simulink model "discrete_angular_rate_subsystem_eso"  (R2019b)
settings: Solver=FixedStepAuto  StartTime=0.0  StopTime=50  FixedStep=1/sim_freq  RelTol=1e-3
values from neighbouring files (symbols this model uses):
  A = diag(ones(length(a)-2,1),1)    [eso_design.m]    (also in eso_design_angular_rate.m = [0 1 0; 0 0 1; 0 0 -500 ]; eso_design_velocity.m = diag(ones(size,1),1); tf2CCF.m; tf2ControlCanonical.m)
  B = zeros(length(a)-1,1)    [eso_design.m]    (also in eso_design_angular_rate.m = [0;B_CONTROL_SYS(end);-500*B_CONTROL_SYS(end)]; eso_design_velocity.m = zeros(size+1,1); tf2CCF.m = zeros(length(A),1))
  C = [1 0 0]    [eso_design_angular_rate.m]    (also in eso_design_velocity.m = zeros(1,size+1); tf2CCF.m = zeros(1,length(b)-1); tf2ControlCanonical.m = zeros(1,length(b)-1))
  L = acker(A',C',poles_eso)'    [eso_design.m]    (also in eso_design_angular_rate.m = [3*wd 3*wd^2 wd^3]'; eso_design_velocity.m = acker(A',C',eso_poles)')
  sim_freq = 1000    [performance_analysis.m]
undefined symbols (not defined in the file or in its folder): dSYS, MC_PITCHRATE_D, MC_PITCHRATE_I, MC_PITCHRATE_P
libraries: simulink x1
settings Model: Creator=henry  LastModifiedBy=henry

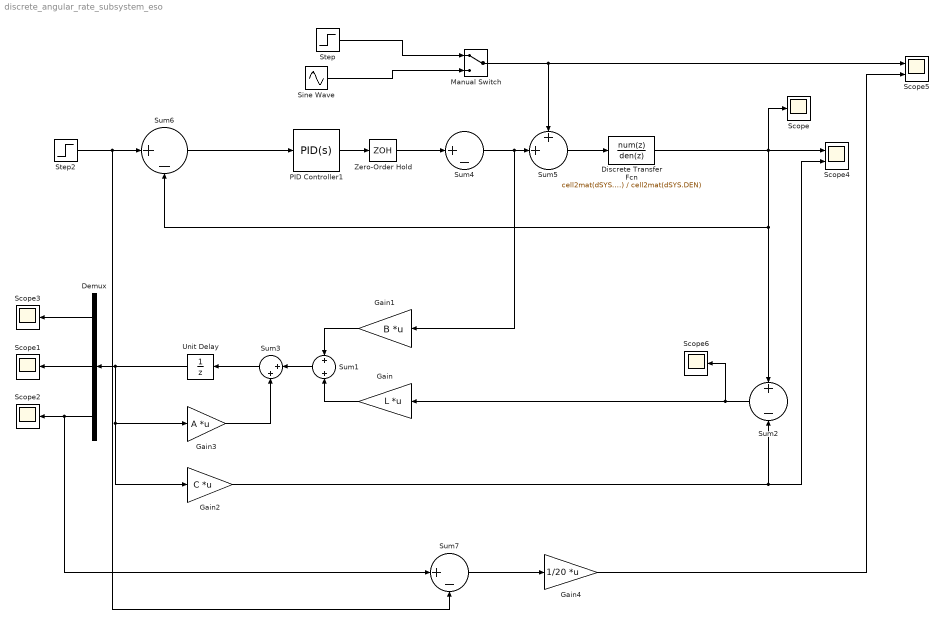
== system discrete_angular_rate_subsystem_eso ==
  Demux : Demux  Outputs=3
  Discrete Transfer Fcn : DiscreteTransferFcn  Numerator=cell2mat(dSYS.NUM)  Denominator=cell2mat(dSYS.DEN)  SampleTime=1/sim_freq
  Gain : Gain  Gain=L  Multiplication=Matrix(K*u)
  Gain1 : Gain  Gain=B  Multiplication=Matrix(K*u)
  Gain2 : Gain  Gain=C  Multiplication=Matrix(K*u)
  Gain3 : Gain  Gain=A  Multiplication=Matrix(K*u)
  Gain4 : Gain  Gain=1/20  Multiplication=Matrix(K*u)
  Manual Switch : ManualSwitch
  PID Controller1 : simulink/Continuous/PID Controller  Controller=PID  Form=Ideal  TimeDomain=Continuous-time  SampleTime=-1  IntegratorMethod=Forward Euler  FilterMethod=Forward Euler  ControllerParametersSource=internal  P=MC_PITCHRATE_P  I=MC_PITCHRATE_I  D=MC_PITCHRATE_D  UseFilter=on  N=100  TunerSelectOption=Transfer Function Based (PID Tuner App)  InitialConditionSource=internal  InitialConditionForIntegrator=0  InitialConditionForFilter=0  DifferentiatorICPrevScaledInput=0  ExternalReset=none  TrackingMode=off  Kt=1  LimitOutput=off  UpperSaturationLimit=inf  LowerSaturationLimit=-inf  LinearizeAsGain=on  AntiWindupMode=none  Kb=1  POutMin=[]  POutMax=[]  IOutMin=[]  IOutMax=[]  DOutMin=[]  DOutMax=[]  NOutMin=[]  NOutMax=[]  SumOutMin=[]  SumOutMax=[]  SaturationOutMin=[]  SaturationOutMax=[]  PParamMin=[]  PParamMax=[]  IParamMin=[]  IParamMax=[]  DParamMin=[]  DParamMax=[]  NParamMin=[]  NParamMax=[]  KbParamMin=[]  KbParamMax=[]  KtParamMin=[]  KtParamMax=[]  KbOutMin=[]  KbOutMax=[]  KtOutMin=[]  KtOutMax=[]  IntegratorOutMin=[]  IntegratorOutMax=[]  FilterOutMin=[]  FilterOutMax=[]  SumI1OutMin=[]  SumI1OutMax=[]  SumI2OutMin=[]  SumI2OutMax=[]  SumI3OutMin=[]  SumI3OutMax=[]  SumI4OutMin=[]  SumI4OutMax=[]  SumDOutMin=[]  SumDOutMax=[]  DifferentiatorOutMin=[]  DifferentiatorOutMax=[]  FilterDiffOutCoefMin=[]  FilterDiffOutCoefMax=[]  ReciprocalOutMin=[]  ReciprocalOutMax=[]  SumDenOutMin=[]  SumDenOutMax=[]  SumNumOutMin=[]  SumNumOutMax=[]  DivideOutMin=[]  DivideOutMax=[]  IntegratorContinuousStateAttributes=''  IntegratorStateMustResolveToSignalObject=off  IntegratorRTWStateStorageClass=Auto  FilterContinuousStateAttributes=''  FilterStateMustResolveToSignalObject=off  FilterRTWStateStorageClass=Auto  ParallelPVariant=Passthrough  IdealPVariant=InternalParameters  IVariant=InternalParameters  DVariant=InternalParameters  IntegratorVariant=Continuous  SatVariant=Disabled  AWVariant=Passthrough  PCopyVariant=Disabled  TRVariant=Disabled  FdbkBlocksVariant=Forward  IdealPFdbkVariant=Disabled  SatFdbkVariant=Disabled  DerivativeFilterVariant=ContFilter  NVariant=InternalParameters  NCopyVariant=Disabled  FilterICVariant=InternalICsFilter  IntegratorICVariant=InternalICs  ExternalResetVariant=Disabled  TRSumVariant=Passthrough  SumFdbkVariant=Disabled  SumVariant=Sum_PID
  Scope{,1..3,6} (5 alike) : Scope
  Scope4 : Scope  NumInputPorts=2
  Scope5 : Scope  NumInputPorts=2
  Sine Wave : Sin  Amplitude=0.1  Frequency=2  SampleTime=0
  Step : Step  Time=5  After=0.5  SampleTime=0
  Step2 : Step  After=2  SampleTime=0
  Sum1 : Sum  Inputs=+|+
  Sum2 : Sum  Inputs=+|-
  Sum3 : Sum  Inputs=|++
  Sum4 : Sum  Inputs=|+-
  Sum5 : Sum  Inputs=++|
  Sum6 : Sum  Inputs=|+-
  Sum7 : Sum  Inputs=|+-
  Unit Delay : UnitDelay  SampleTime=-1  HasFrameUpgradeWarning=on
  Zero-Order Hold : ZeroOrderHold  SampleTime=1/sim_freq
  wires:
  Sum6/1 -> PID Controller1/1
  Step2/1 -> Sum7/2, Sum6/1
  Demux/2 -> Scope1/1
  Gain/1 -> Sum1/2
  Demux/1 -> Scope3/1
  Gain1/1 -> Sum1/1
  Gain3/1 -> Sum3/2
  Sum1/1 -> Sum3/1
  Sum3/1 -> Unit Delay/1
  Unit Delay/1 -> Gain3/1, Gain2/1, Demux/1
  Sum2/1 -> Scope6/1, Gain/1
  Sum5/1 -> Discrete Transfer Fcn/1
  Demux/3 -> Sum7/1, Scope2/1
  PID Controller1/1 -> Zero-Order Hold/1
  Gain2/1 -> Sum2/2, Scope4/2
  Discrete Transfer Fcn/1 -> Sum2/1, Sum6/2, Scope/1, Scope4/1
  Sum4/1 -> Gain1/1, Sum5/2
  Gain4/1 -> Scope5/2
  Zero-Order Hold/1 -> Sum4/1
  Sum7/1 -> Gain4/1
  Step/1 -> Manual Switch/1
  Manual Switch/1 -> Sum5/1, Scope5/1
  Sine Wave/1 -> Manual Switch/2
